simulink model "Compare"  (R2020b)
settings: Solver=ode23tb  StartTime=0.0  StopTime=200  RelTol=5e-2
model workspace (MAT data in the model file):
  DownShiftSpeeds = [11.05  11.05  11.05  11.05  11.05  11.05  11.05  11.05  11.05  11.05  11.05  11.05  19.55  25.5  31.45  35.7  35.7; 18.7  18.7  18.7  18.7  19.125  20.48636  21.33636  23.375  27.28636  30.26136  33.827365  38.76136  46.072635  56.1  64.6  73.1  73.1; 28.9  28.9  28.9  28.9  28.9  30.51364  34.51136  41.56364  47.68636  53.377365  58.477365  65.622635  73.525  81.26136  88.48636  115.6  115.6; 38.675  38.675  38.675  38.675  39.43864  42.41364  47.68636  56.43864  65.11136  72.927365  80.497635  90.01364  100.81136  110.672635  122.4  153  153; 51.425  51.425  51.425  51.425  51.76364  55.077365  62.38864  72.422635  83.3  102  136  425  425  425  425  425  425]
  I = 0.25
  Kbr = 1000000
  MGUMaxPower = 50000
  P = 15
  PedalPositions = [0 6.2485 12.4969 18.7454 24.9939 31.2424 37.4908 43.7393 49.9878 56.2363 62.4847 68.7332 74.9817 81.2302 87.4786 93.7271 99.9756]
  SOCmax = 99
  TrqICMax = 175
  TrqMGUMax = 150
  TrqMax = 325
  UpShiftSpeeds = [12.75  12.75  12.75  12.75  12.75  12.75  15.552365  17.08636  18.7  20.227365  23.46136  27.625  31.702365  36.63636  42.5  42.5  42.5; 20.997635  20.997635  20.997635  20.997635  21.927365  24.902365  28.727365  31.78864  35.275  39.697635  46.41136  51.85  59.672635  67.48864  78.2  78.2  78.2; 31.45  31.45  31.45  31.45  34.172635  41.052365  47.175  52.952365  59.5  68  76.5  85  93.5  106.25  119.85  119.85  119.85; 42.16136  42.16136  42.16136  43.947635  47.002365  54.31364  63.325  71.227365  79.222635  88.06136  98.852365  109.052365  118.402365  128.86136  157.25  157.25  157.25; 55.58864  55.58864  55.58864  58.052365  61.53864  72.077365  85.51136  96.81364  255  255  255  255  255  255  255  255  255]
  axle_b = 10
  axle_k = 5000
  bevAxle_wc = 400
  bevNp = 2
  bevNs = 30
  brkTrqMGU = 150
  brkTrqMax = 700
  convAxle_wc = 500
  diffRatio = 3.4
  diffRatio1 = 3.4
  driveshaft_b = 10
  driveshaft_k = 2500
  driveshaft_wc = 500
  engineSpeedPoints_rpm = [750 1053.57142857 1357.14285714 1660.71428571 1964.28571429 2267.85714286 2571.42857143 2875 3178.57142857 3482.14285714 3785.71428571 4089.28571429 4392.85714286 4696.42857143 5000]
  engineTorqueMap_Nm = [-13.6738264269 15.0034460821 26.4289521305 37.8539339756 49.2854604964 60.7146317399 72.0173711595 77.7345012802 77.7345012802 77.7345012802 77.7345012802 77.7345012802 ... (240 elements, 16x15)]
  engineTorquePoints_Nm = [0 15 26.4285714286 37.8571428571 49.2857142857 60.7142857143 72.1428571429 83.5714285714 95 106.428571429 117.857142857 129.285714286 140.714285714 152.142857143 163.571428571 175]
  fuelCapacity = 35
  motorMaxTorqueNm = [500 500 500 500 500 500 416.666666667 357.142857143 312.5 277.777777778 250 227.272727273 208.333333333 192.307692308 178.571428571 166.666666667]
  motorSpeedRadPs = [0 40 80 120 160 200 240 280 320 360 400 440 480 520 560 600]
  tau_IC = 2
  tau_Regen = 1
  vehicleMass = 1500
  wheelRadius = 0.35
libraries: autolibshared x2, pil_lib x1
settings Model: Creator=ivane  LastModifiedBy=rubbi
settings OptimizationCC: OptimizeBlockIOStorage=off
settings RTWCC: BuildConfiguration=Debug
settings CodeAppCC: ForceParamTrailComments=on  MATLABSourceComments=on

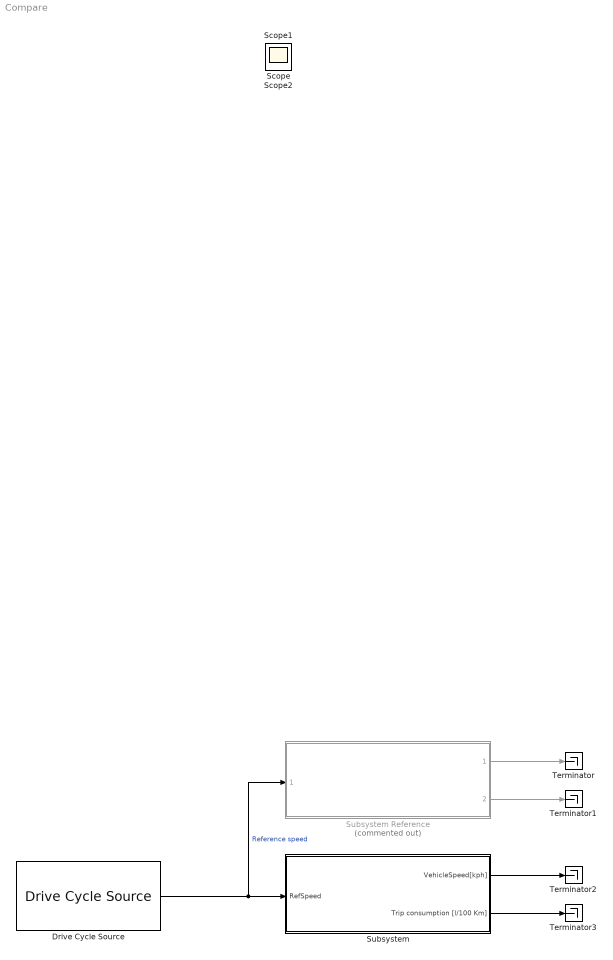
== system Compare ==
  Drive Cycle Source : autolibshared/Drive Cycle Source  cycleVar=Workspace variable  wsVar=WLTP_class_3  fileVar=cycleFTP75.mat  tfinal="1800  seconds"  cycleRepeat=off  outAccPort=off  outGearPort=off  gearList=No gear data  t_wot1=5  xdot_woto=0  xdot_wot1=30  t_wot2=20  xdot_wot2=0  t_wotend=30  srcUnit=km/h  outUnit=km/h  srcAccUnit=m/s/s  outAccUnit=m/s^2  dt=0  aMode=1  faultOption=off  velBnd=2  velBndUnit=mph  inUnit=m/s  timeBnd=1  failOption=off  stopSim=off  maxFaultCnt=10  maxFaultTime=2  maxTotFaultTime=15  traceOption=off  dtTrace=1  traceWindow=10  lastDCname=Custom Data Set 1  lastOutUnit=mph  lastDT=0  lastTB=1  lastSB=2  forceCalcBound=off
      settings: SourceProductBaseCode=PW,MT,UV,VE,VP
  Subsystem : Subsystem
  Subsystem Reference : Subsystem  Commented=on  ReferencedSubsystem=standardVehicle
  Terminator{,1..3} (4 alike) : Terminator
  Scope : Scope
  Scope1 : Scope
  Scope2 : Scope
  wires:
  Drive Cycle Source/1 -> Subsystem Reference/1, Subsystem/1(RefSpeed)  "Reference speed"
  Subsystem Reference/1 -> Terminator/1
  Subsystem Reference/2 -> Terminator1/1
  Subsystem/2(Trip consumption [l/100 Km]) -> Terminator3/1
  Subsystem/1(VehicleSpeed[kph]) -> Terminator2/1

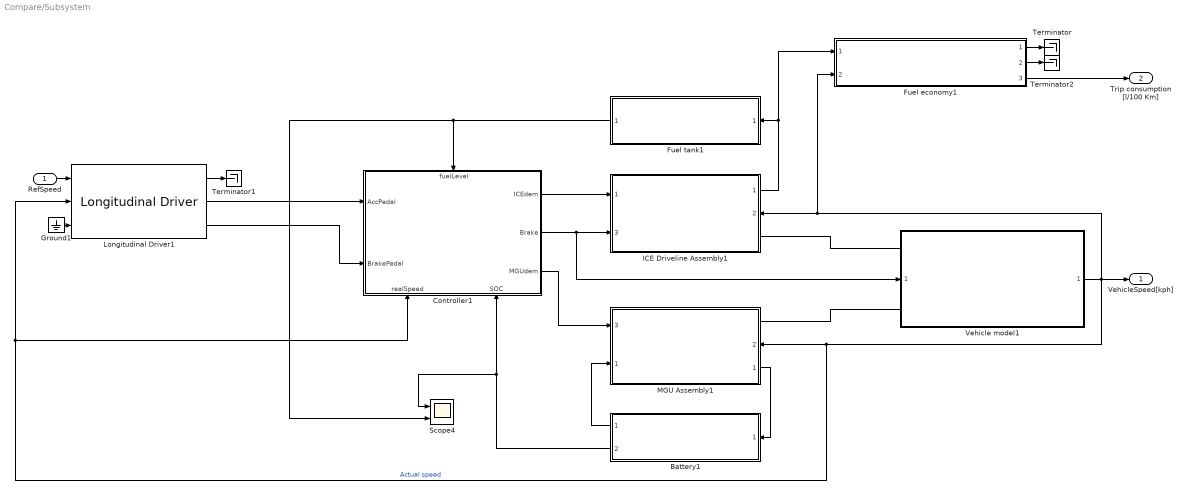
== system Compare/Subsystem ==
  RefSpeed : Inport
  Battery1 : Subsystem  ReferencedSubsystem=Battery
      settings: PortSchema="{\"entries\":[{\"content\":{\"sides\":[{\"content\":{\"connectorIds\":[\"Out1\",\"Out2\"]},\"type\":\"ConnectorPlacement.EquallySpacedRectSide\",\"uuid\":\"62c661fb-2963-4729-8409-c11ca18452bb\"},{\"content\":{\"connectorIds\":[\"In1\"],\"side\":\"RIGHT\"},\"type\":\"ConnectorPlacement.EquallySpacedRectSide\",\"uuid\":\"8d8a0df4-31a2-4844-b6e4-fdfd8750374f\"},{\"content\":{\"connectorIds\":[],\"side\":\"TOP\"},\"type\":\"ConnectorPlacement.EquallySpacedRectSide\",\"uuid\":\"345d14b7-5d59-4ed6-ba31-c78cc2155fc5\"},{\"content\":{\"connectorIds\":[],\"side\":\"HIDDEN\"},\"type\":\"ConnectorPlacement.EquallySpacedRectSide\",\"uuid\":\"be681e4d-0788-4d60-9432-78c6b7c184d6\"}]},\"type\":\"ConnectorPlacement.EquallySpacedConnector\",\"uuid\":\"76d22945-58a4-4f01-9ad4-fc5d192e1319\"}],\"packageUris\":[\"http://schema.mathworks.com/mf0/Connector/R2020b\"],\"version\":\"1.0\"}"
  Controller1 : Subsystem  DialogController=pil_create_dialog  LoadFcn=|
      | try
      |    if ~strcmp(rtw.pil.getPILVersion, '9.9 (R2020b)_14')
      |       set_param(gcb, 'DialogController', '');
      |       set_param(gcb, 'DialogControllerArgs', '');
      |    end
      | catch e
      |       set_param(gcb, 'DialogController', '');
      |       set_param(gcb, 'DialogControllerArgs', '');
      | end
      mask help: PIL:pil:XILBlockMaskDesc
      settings: PortSchema="{\"entries\":[{\"content\":{\"sides\":[{\"content\":{\"connectorIds\":[\"In1\",\"In2\"]},\"type\":\"ConnectorPlacement.EquallySpacedRectSide\",\"uuid\":\"da5a9760-f191-46b2-9412-225508306177\"},{\"content\":{\"connectorIds\":[\"Out1\",\"Out2\",\"Out3\"],\"side\":\"RIGHT\"},\"type\":\"ConnectorPlacement.EquallySpacedRectSide\",\"uuid\":\"51ee291c-9e13-4f9e-bc88-42dd36fcbd58\"},{\"content\":{\"connectorIds\":[\"In3\"],\"side\":\"TOP\"},\"type\":\"ConnectorPlacement.EquallySpacedRectSide\",\"uuid\":\"7cb132c6-2afa-42fb-93bc-2c05524d5014\"},{\"content\":{\"connectorIds\":[\"In4\",\"In5\"],\"side\":\"BOTTOM\"},\"type\":\"ConnectorPlacement.EquallySpacedRectSide\",\"uuid\":\"eca246fa-4264-454d-a17a-e551cde90ce4\"},{\"content\":{\"connectorIds\":[],\"side\":\"HIDDEN\"},\"type\":\"ConnectorPlacement.EquallySpacedRectSide\",\"uuid\":\"02d58808-80ce-4ef1-80f9-06eee9ea1ac6\"}]},\"type\":\"ConnectorPlacement.EquallySpacedConnector\",\"uuid\":\"787de183-772d-42fe-8514-c26c1daff49c\"}],\"packageUris\":[\"http://schema.mathworks.com/mf0/Connector/R2020b\"],\"version\":\"1.0\"}"
      mask Display: disp('SIL');
  Fuel economy1 : Subsystem  ReferencedSubsystem=Fuel_economy
  Fuel tank1 : Subsystem  ReferencedSubsystem=fuelTank
  Ground1 : Ground
  ICE Driveline Assembly1 : Subsystem  ReferencedSubsystem=IC_Driveline
      settings: PortSchema="{\"entries\":[{\"content\":{\"sides\":[{\"content\":{\"connectorIds\":[\"In1\",\"In3\"]},\"type\":\"ConnectorPlacement.EquallySpacedRectSide\",\"uuid\":\"d2a2af2f-0810-46c5-a89d-1fb3bffb58b0\"},{\"content\":{\"connectorIds\":[\"Out1\",\"In2\",\"RConn1\"],\"side\":\"RIGHT\"},\"type\":\"ConnectorPlacement.EquallySpacedRectSide\",\"uuid\":\"5d91c2bd-bc93-425c-9733-5ba49e3ee9da\"},{\"content\":{\"connectorIds\":[],\"side\":\"TOP\"},\"type\":\"ConnectorPlacement.EquallySpacedRectSide\",\"uuid\":\"30272aa7-5431-486b-ba2d-786d8a62fe2e\"},{\"content\":{\"connectorIds\":[],\"side\":\"HIDDEN\"},\"type\":\"ConnectorPlacement.EquallySpacedRectSide\",\"uuid\":\"f07e1d6c-3558-4c7b-844c-ecaea33e0b73\"}]},\"type\":\"ConnectorPlacement.EquallySpacedConnector\",\"uuid\":\"e11bd347-ea62-4e54-9941-5a9032f6c7d6\"}],\"packageUris\":[\"http://schema.mathworks.com/mf0/Connector/R2020b\"],\"version\":\"1.0\"}"
  Longitudinal Driver1 : autolibshared/Longitudinal Driver  extAccelOvr=off  extDecelOvr=off  extAccelHld=off  extDecelHld=off  extAccelZero=off  extDecelZero=off  cntrlType=PI  shftType=None  velUnits=km/h  gearOut=off  Kp=15  Ki=0.5  Kff=0  Kg=0  VehVelVec=[0 100]  KffVec=[.1 .1]  KpVec=[10 10]  KiVec=[5 5]  KgVec=[0 0]  m=1500  Kpt=3000  tau=.1  L=2  aR=200  bR=2.5  cR=.5  g=9.81  vnom=100  Kaw=0  tauerr=.0  tauPt=2  GearInit=0  tShift=.1  pdlVec=[0.1 0.4 0.5 0.9]  upShftTbl=[-1 12.9375 26.4375 39.9375 51.18749999999999 62.4375 72.84375 83.25;-1 16.3125 29.8125 43.3125 54.5624 65.8125 76.78125 87.75;-1 19.6875 33.1875 46.68749999999999 57.9375 69.1875 80.71875 92.25;-1 33 52.5 77.25 100.5 138.75 161.875 185]  dwnShftTbl=[1 9.5625 23.0625 36.5625 47.8125 59.0625 68.90625 78.75;1 12.9375 26.4375 39.9375 51.18749999999999 62.4375 72.84375 83.25;1 16.3125 29.8125 43.3125 54.562499 65.8125 76.78125 87.75;1 19.6875 33.1875 46.68749999999999 57.9375 69.1875 80.71875 92.25]  tClutch=.5  tRev=.5  tPark=120  aMode=1  UpGearVec="[0  1  2  3  4  5  6  7]"  DownGearVec="[1  2  3  4  5  6  7  8]"
      settings: SourceProductBaseCode=PW,MT,UV,VE,VP
  MGU Assembly1 : Subsystem  ReferencedSubsystem=MGU
      settings: PortSchema="{\"entries\":[{\"content\":{\"sides\":[{\"content\":{\"connectorIds\":[\"In3\",\"In1\"]},\"type\":\"ConnectorPlacement.EquallySpacedRectSide\",\"uuid\":\"d2a2af2f-0810-46c5-a89d-1fb3bffb58b0\"},{\"content\":{\"connectorIds\":[\"RConn1\",\"In2\",\"Out1\"],\"side\":\"RIGHT\"},\"type\":\"ConnectorPlacement.EquallySpacedRectSide\",\"uuid\":\"5d91c2bd-bc93-425c-9733-5ba49e3ee9da\"},{\"content\":{\"connectorIds\":[],\"side\":\"TOP\"},\"type\":\"ConnectorPlacement.EquallySpacedRectSide\",\"uuid\":\"30272aa7-5431-486b-ba2d-786d8a62fe2e\"},{\"content\":{\"connectorIds\":[],\"side\":\"HIDDEN\"},\"type\":\"ConnectorPlacement.EquallySpacedRectSide\",\"uuid\":\"f07e1d6c-3558-4c7b-844c-ecaea33e0b73\"}]},\"type\":\"ConnectorPlacement.EquallySpacedConnector\",\"uuid\":\"e11bd347-ea62-4e54-9941-5a9032f6c7d6\"}],\"packageUris\":[\"http://schema.mathworks.com/mf0/Connector/R2020b\"],\"version\":\"1.0\"}"
  Scope4 : Scope  NumInputPorts=2
  Terminator : Terminator
  Terminator1 : Terminator
  Terminator2 : Terminator
  Vehicle model1 : Subsystem  ReferencedSubsystem=vehicleModel
      settings: PortSchema="{\"entries\":[{\"content\":{\"sides\":[{\"content\":{\"connectorIds\":[\"LConn1\",\"In1\",\"LConn2\"]},\"type\":\"ConnectorPlacement.EquallySpacedRectSide\",\"uuid\":\"297baffa-e0bc-4afe-8d3b-fef71b7412b4\"},{\"content\":{\"connectorIds\":[\"Out1\"],\"side\":\"RIGHT\"},\"type\":\"ConnectorPlacement.EquallySpacedRectSide\",\"uuid\":\"8a12a35b-b522-4ba0-9ba0-852b497f573e\"},{\"content\":{\"connectorIds\":[],\"side\":\"TOP\"},\"type\":\"ConnectorPlacement.EquallySpacedRectSide\",\"uuid\":\"b4b51f6d-39af-472b-beff-f9410fe777e8\"},{\"content\":{\"connectorIds\":[],\"side\":\"HIDDEN\"},\"type\":\"ConnectorPlacement.EquallySpacedRectSide\",\"uuid\":\"ccc4846e-18b0-46b1-8b77-dbf40ce11e43\"}]},\"type\":\"ConnectorPlacement.EquallySpacedConnector\",\"uuid\":\"224bfd92-7422-4b82-8ee3-7d4031b335e8\"}],\"packageUris\":[\"http://schema.mathworks.com/mf0/Connector/R2020b\"],\"version\":\"1.0\"}"
  VehicleSpeed[kph] : Outport
  Trip consumption [l/100 Km] : Outport  Port=2
  wires:
  Controller1/3(MGUdem) -> MGU Assembly1/3
  Battery1/2 -> Scope4/1, Controller1/5(SOC)
  Ground1/1 -> Longitudinal Driver1/3
  Vehicle model1/1 -> VehicleSpeed[kph]/1, MGU Assembly1/2, Controller1/4(realSpeed), Longitudinal Driver1/2, Fuel economy1/2, ICE Driveline Assembly1/2  "Actual speed"
  Fuel tank1/1 -> Scope4/2, Controller1/3(fuelLevel)
  Longitudinal Driver1/1 -> Terminator1/1
  MGU Assembly1/1 -> Battery1/1
  Controller1/2(Brake) -> Vehicle model1/1, ICE Driveline Assembly1/3
  ICE Driveline Assembly1/1 -> Fuel economy1/1, Fuel tank1/1
  RefSpeed/1 -> Longitudinal Driver1/1
  Controller1/1(ICEdem) -> ICE Driveline Assembly1/1
  Longitudinal Driver1/2 -> Controller1/1(AccPedal)
  Battery1/1 -> MGU Assembly1/1
  Longitudinal Driver1/3 -> Controller1/2(BrakePedal)
  Fuel economy1/3 -> Trip consumption [l/100 Km]/1
  Fuel economy1/1 -> Terminator/1
  Fuel economy1/2 -> Terminator2/1
  connections:
  ICE Driveline Assembly1/RConn1 -- Vehicle model1/LConn1
  Vehicle model1/LConn2 -- MGU Assembly1/RConn1

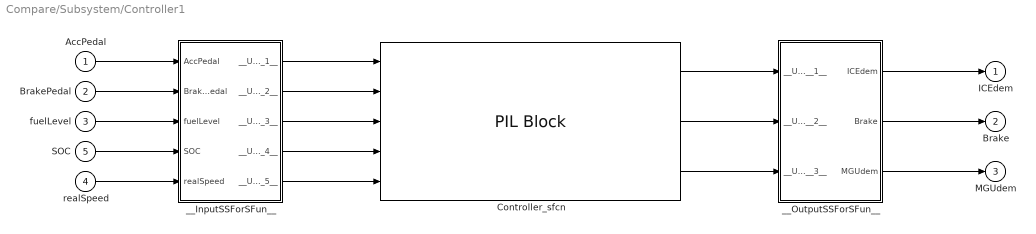
== system Compare/Subsystem/Controller1 ==
  AccPedal : Inport
  BrakePedal : Inport  Port=2
  fuelLevel : Inport  Port=3
  realSpeed : Inport  Port=4
  SOC : Inport  Port=5
  Controller_sfcn : pil_lib/PIL Block  SimulationMode=SIL  IsTopModelPIL=off  CodeDir=C:\Users\rubbi\Desktop\CoDeAS\hybrid-controller\Hybrid-controller\Code\Controller_ert_rtw  AnchorDir=C:\Users\rubbi\Desktop\CoDeAS\hybrid-controller\Hybrid-controller\Code  ConfigName=Software-in-the-Loop (SIL)  XrelIsTopModelCode=on  XrelIsReusable=off  XrelDWorkNames={}  XrelDWorkTypes={}  XrelModelArgVals={}  XrelOrderedParamNames={}
      settings: SourceProductBaseCode=RT
  __InputSSForSFun__ : Subsystem
  __OutputSSForSFun__ : Subsystem
  ICEdem : Outport
  Brake : Outport  Port=2
  MGUdem : Outport  Port=3
  wires:
  AccPedal/1 -> __InputSSForSFun__/1(AccPedal)
  BrakePedal/1 -> __InputSSForSFun__/2(BrakePedal)
  fuelLevel/1 -> __InputSSForSFun__/3(fuelLevel)
  SOC/1 -> __InputSSForSFun__/4(SOC)
  realSpeed/1 -> __InputSSForSFun__/5(realSpeed)
  __InputSSForSFun__/1(__UniqueOutportName__1__) -> Controller_sfcn/1
  __InputSSForSFun__/2(__UniqueOutportName__2__) -> Controller_sfcn/2
  __InputSSForSFun__/3(__UniqueOutportName__3__) -> Controller_sfcn/3
  __InputSSForSFun__/4(__UniqueOutportName__4__) -> Controller_sfcn/4
  __InputSSForSFun__/5(__UniqueOutportName__5__) -> Controller_sfcn/5
  Controller_sfcn/1 -> __OutputSSForSFun__/1(__UniqueInportName__1__)
  Controller_sfcn/2 -> __OutputSSForSFun__/2(__UniqueInportName__2__)
  Controller_sfcn/3 -> __OutputSSForSFun__/3(__UniqueInportName__3__)
  __OutputSSForSFun__/1(ICEdem) -> ICEdem/1
  __OutputSSForSFun__/2(Brake) -> Brake/1
  __OutputSSForSFun__/3(MGUdem) -> MGUdem/1

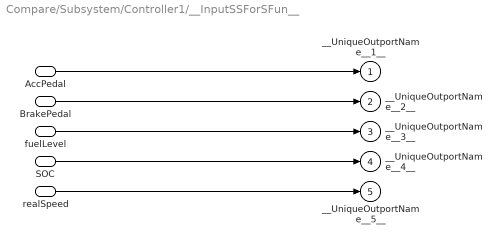
== system Compare/Subsystem/Controller1/__InputSSForSFun__ ==
  AccPedal : Inport
  BrakePedal : Inport  Port=2
  fuelLevel : Inport  Port=3
  SOC : Inport  Port=4
  realSpeed : Inport  Port=5
  __UniqueOutportName__1__ : Outport
  __UniqueOutportName__2__ : Outport  Port=2
  __UniqueOutportName__3__ : Outport  Port=3
  __UniqueOutportName__4__ : Outport  Port=4
  __UniqueOutportName__5__ : Outport  Port=5
  wires:
  AccPedal/1 -> __UniqueOutportName__1__/1
  BrakePedal/1 -> __UniqueOutportName__2__/1
  fuelLevel/1 -> __UniqueOutportName__3__/1
  SOC/1 -> __UniqueOutportName__4__/1
  realSpeed/1 -> __UniqueOutportName__5__/1

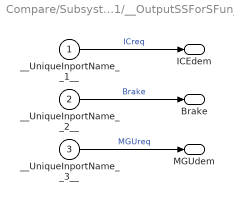
== system Compare/Subsystem/Controller1/__OutputSSForSFun__ ==
  __UniqueInportName__1__ : Inport
  __UniqueInportName__2__ : Inport  Port=2
  __UniqueInportName__3__ : Inport  Port=3
  ICEdem : Outport
  Brake : Outport  Port=2
  MGUdem : Outport  Port=3
  wires:
  __UniqueInportName__1__/1 -> ICEdem/1  "ICreq"
  __UniqueInportName__2__/1 -> Brake/1  "Brake"
  __UniqueInportName__3__/1 -> MGUdem/1  "MGUreq"
